simulink model "paraglider_sim_model"  (R2016a)
settings: Solver=VariableStepAuto  StartTime=0.0  StopTime=10.0  RelTol=1e-3
InitFcn:
  | addpath('..');
settings Model: Creator=AkhramovichSA  LastModifiedBy=AkhramovichSA

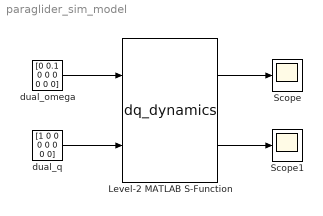
== system paraglider_sim_model ==
  Level-2 MATLAB S-Function : M-S-Function  FunctionName=dq_dynamics
  Scope : Scope
  Scope1 : Scope
  dual_omega : Constant  Value=[0 0.1 0 0 0 0 0 0]
  dual_q : Constant  Value=[1 0 0 0 0 0 0 0]
  wires:
  dual_omega/1 -> Level-2 MATLAB S-Function/1
  dual_q/1 -> Level-2 MATLAB S-Function/2
  Level-2 MATLAB S-Function/1 -> Scope/1
  Level-2 MATLAB S-Function/2 -> Scope1/1
